simulink model "PGS_STD_SINV_2STAGE_MODEL_RLOAD"  (R2024b)
settings: Solver=VariableStepAuto  StartTime=0.0  StopTime=2.0  RelTol=1e-3
PostLoadFcn:
  | gmp_model_file=get_param(bdroot,'FileName'); if isempty(gmp_model_file), error('GMP:SINV:ModelPath', 'The SINV model must be saved before SDPE initialization.'); end; gmp_model_dir=fileparts(gmp_model_file); run(fullfile(gmp_model_dir,'sdpe_mgr','ctrl_settings_matlab_init.m')); gmp_matlab_release=matlabRelease; addpath(fullfile(gmp_model_dir,'..','..','..','..','..','slib','install_path',gmp_matlab_release.Release,'src')); clear gmp_model_file gmp_model_dir gmp_matlab_release;
InitFcn:
  | gmp_model_file=get_param(bdroot,'FileName'); if isempty(gmp_model_file), error('GMP:SINV:ModelPath', 'The SINV model must be saved before SDPE initialization.'); end; gmp_model_dir=fileparts(gmp_model_file); run(fullfile(gmp_model_dir,'sdpe_mgr','ctrl_settings_matlab_init.m')); gmp_matlab_release=matlabRelease; addpath(fullfile(gmp_model_dir,'..','..','..','..','..','slib','install_path',gmp_matlab_release.Release,'src')); clear gmp_model_file gmp_model_dir gmp_matlab_release;
undefined symbols (not defined in the file or in its folder): CTRL_AC_CURRENT_BIAS, CTRL_AC_CURRENT_SENSITIVITY, CTRL_AC_INDUCTANCE, CTRL_AC_RESISTANCE, CTRL_AC_VOLTAGE_BIAS, CTRL_AC_VOLTAGE_SENSITIVITY, CTRL_ADC_RESOLUTION, CTRL_ADC_VOLTAGE_REF, CTRL_DC_VOLTAGE_BIAS, CTRL_DC_VOLTAGE_SENSITIVITY, CTRL_DCBUS_VOLTAGE, CTRL_PWM_CMP_MAX, CTRL_PWM_DEADBAND_CMP, SINV_CURRENT_AMPLIFIER_GAIN, SINV_CURRENT_SHUNT_OHM, SINV_DC_CAP_EPR_OHM, SINV_DC_CAP_ESR_OHM, SINV_DC_CAPACITANCE_F, SINV_FILTER_CAP_EPR_OHM, SINV_FILTER_CAP_ESR_OHM, SINV_FILTER_CAPACITANCE_F, SINV_MODEL_DIODE_RON, SINV_MODEL_DIODE_VF, SINV_MODEL_MOSFET_RON, SINV_PWM_FREQUENCY_HZ, SINV_RLOAD_OHM, SINV_SENSOR_FILTER_HZ
libraries: spsSeriesRLCBranchLib x13, spsVoltageMeasurementLib x7, spsSecondOrderFilterLib x6, gmp_peripheral_utilities x3, spsMosfetLib x2, spsCurrentMeasurementLib x2, gmp_fp_utilities x1, gmp_sil_core_pack x1, spsControlledVoltageSourceLib x1, spspowerguiLib x1
(part 1 of 2)
settings Model: SimulationMode=accelerator  Creator=javnson  LastModifiedBy=javnson

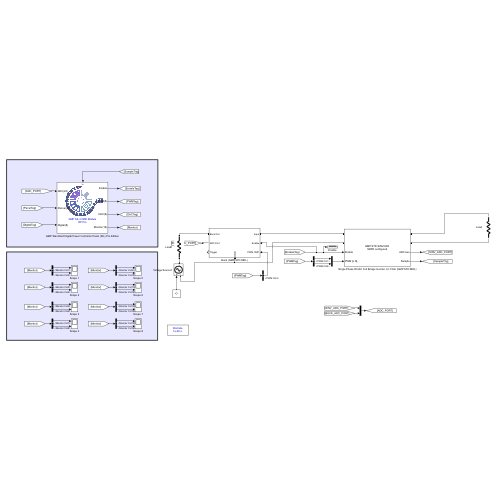
[thumbnail: Simulink's stored preview of the top-level diagram]
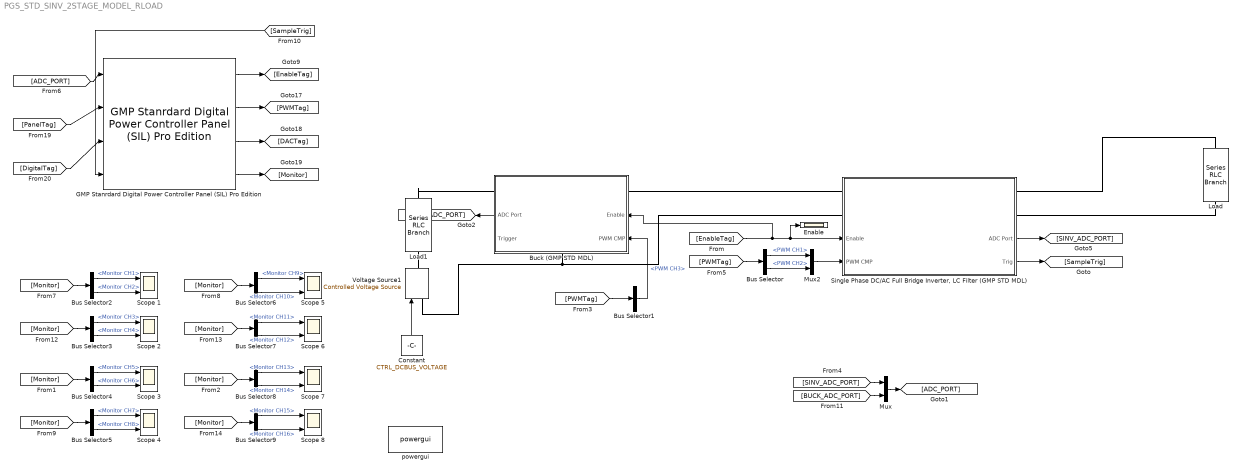
== system PGS_STD_SINV_2STAGE_MODEL_RLOAD ==
  Buck (GMP STD MDL) : Subsystem  mask(GMP Standard Digital Power Submodule - Buck){R_mosfet_on=4.6e-3, Lon=0, Rd=0.01, Vf=0.5, Rs=1e5, Cs=inf, L_main=680e-6, L_ESR=0.05, Cin_main=680e-6, Cin_ESR=0.09, Cout_main=680e-6, Cout_ESR=0.09, fswitch=20e3, CMP_MAX=4200-1, Deadband_Upper=80, Deadband_Lower=80, phase_shift=0, ADC_Resolution=12, Voltage_Gain=2.2/202.2, VOLTAGE_ADC_REFERENCE=2.5, VOLTAGE_ADC_BIAS=0.9966, VOLTAGE_ADC_INIT=0, VOLTAGE_ADC_CUT_FREQ=1.5e3, Current_Gain=0.005*20, CURRENT_ADC_REFERENCE=2.5, CURRENT_ADC_BIAS=0.9, CURRENT_ADC_INIT=0}
      mask prompts: ADC_Resolution "ADC_BIT:"; Voltage_Gain "ADC_GAIN:"; VOLTAGE_ADC_REFERENCE "ADC_REFERENCE:"; VOLTAGE_ADC_BIAS "ADC_BIAS:"; VOLTAGE_ADC_INIT "ADC_INIT:"; VOLTAGE_ADC_CUT_FREQ "cut_frequency:"; Current_Gain "ADC_GAIN:"; CURRENT_ADC_REFERENCE "ADC_REFERENCE:"; CURRENT_ADC_BIAS "ADC_BIAS:"; CURRENT_ADC_INIT "ADC_INIT:"
      mask help: This is a Standard Buck Module.
      settings: PortSchema="{\"entries\":[{\"content\":{\"sides\":[{\"content\":{\"connectorIds\":[\"LConn1\",\"In1\",\"In2\"]},\"type\":\"ConnectorPlacement.EquallySpacedRectSide\",\"uuid\":\"14f7e26c-4d08-496b-8d9c-39acdf23712e\"},{\"content\":{\"connectorIds\":[\"RConn1\",\"Out1\",\"Out2\"],\"side\":\"RIGHT\"},\"type\":\"ConnectorPlacement.EquallySpacedRectSide\",\"uuid\":\"c4fec36d-dc89-4255-810a-778c215f41bb\"},{\"content\":{\"side\":\"TOP\"},\"type\":\"ConnectorPlacement.EquallySpacedRectSide\",\"uuid\":\"1b2864bd-03e2-4902-8158-79673144629a\"},{\"content\":{\"connectorIds\":[\"RConn2\"],\"side\":\"BOTTOM\"},\"type\":\"ConnectorPlacement.EquallySpacedRectSide\",\"uuid\":\"d3456d19-e299-4c35-abfd-6fb99773e971\"}]},\"type\":\"ConnectorPlacement.EquallySpacedConnector\",\"uuid\":\"dbc738c4-c361-40e9-b3e6-9b32447065a0\"}],\"packageUris\":[\"http://schema.mathworks.com/mf0/Connector/R2020b\"],\"version\":\"1.0\"}"
      mask DialogControl ParameterGroupVar Prompt: 参数
      mask DialogControl Container4 Prompt: Component Parameters
      mask DialogControl Container7 Prompt: MOSFET
      mask DialogControl Control8 Prompt: Rds(on), unit Ohm
      mask DialogControl Control9 Prompt: Internal diode inducctance, unit H
      mask DialogControl Control10 Prompt: Internal diode resistance Rd, unit Ohm
      mask DialogControl Control11 Prompt: Internal diode forward voltage Vf, unit V
      mask DialogControl Control12 Prompt: Snubber resistance Rs, unit ohm
      mask DialogControl Control13 Prompt: Snubber Capacitance Cs, unit F
      mask DialogControl Container8 Prompt: LC Filter
      mask DialogControl Control25 Prompt: main inductance (H):
      mask DialogControl Control26 Prompt: Inductance ESR (Ohm):
      mask DialogControl Control27 Prompt: Main Input Capacitor (F):
      mask DialogControl Control28 Prompt: Input Capcitor ESR (Ohm):
      mask DialogControl Control29 Prompt: Main Output Capacitor (F):
      mask DialogControl Control30 Prompt: Output Capcitor ESR (Ohm):
      mask DialogControl Container5 Prompt: PWM Parameers
      mask DialogControl Control3 Prompt: PWM Frequency (Hz):
      mask DialogControl Control4 Prompt: Full Scale PWM Compare value:
      mask DialogControl Control6 Prompt: (whole period is 2 * CMP_MAX ticks)
      mask DialogControl Control5 Prompt: Deadband Range Set (CMP Value):
      mask DialogControl Control7 Prompt: Single side deadband time: DEADBAND_CMP/2/CMP_MAX/fswitch
      mask DialogControl Control2 Prompt: Initial Phase Shift, unit rad
      mask DialogControl Container6 Prompt: ADC Parameters
      mask DialogControl Container9 Prompt: ADC Device
      mask DialogControl Control14 Prompt: ADC resolution:
      mask DialogControl Container10 Prompt: Voltage Sensor
      mask DialogControl Control15 Prompt: ADC Voltage Gain (Scale Factor):
      mask DialogControl Control16 Prompt: ADC reference Voltage(V)
      mask DialogControl Control Prompt: ADC Bias Voltage(V)
      mask DialogControl Control18 Prompt: ADC Initial Voltage Output (V):
      mask DialogControl Control19 Prompt: Voltage Filter cut frequency (Hz):
      mask DialogControl Control20 Prompt: Generally, this value less than switch frequency / 10, greater than motor normal frequency * 3
      mask DialogControl Container11 Prompt: Current Sensor
      mask DialogControl Control21 Prompt: ADC Current Gain (Scale Factor):
      mask DialogControl Control22 Prompt: ADC reference Current(A), ADC full scale current (when gain = 1)
      mask DialogControl Control23 Prompt: ADC Bias Current(A)
      mask DialogControl Control24 Prompt: ADC initial Current Output(A)
  Bus Selector : BusSelector  OutputSignals=PWM CH1,PWM CH2
  Bus Selector1 : BusSelector  OutputSignals=PWM CH3
  Bus Selector2 : BusSelector  OutputSignals=Monitor CH1,Monitor CH2
  Bus Selector3 : BusSelector  OutputSignals=Monitor CH3,Monitor CH4
  Bus Selector4 : BusSelector  OutputSignals=Monitor CH5,Monitor CH6
  Bus Selector5 : BusSelector  OutputSignals=Monitor CH7,Monitor CH8
  Bus Selector6 : BusSelector  OutputSignals=Monitor CH9,Monitor CH10
  Bus Selector7 : BusSelector  OutputSignals=Monitor CH11,Monitor CH12
  Bus Selector8 : BusSelector  OutputSignals=Monitor CH13,Monitor CH14
  Bus Selector9 : BusSelector  OutputSignals=Monitor CH15,Monitor CH16
  Constant : Constant  Value=CTRL_DCBUS_VOLTAGE
  Enable : Scope
  GMP Stanrdard Digital Power Controller Panel (SIL) Pro Edition : gmp_sil_core_pack/GMP Stanrdard Digital Power Controller Panel (SIL) Pro Edition
      settings: SourceProductName=GMP SIL Core Utilities
  Load : spsSeriesRLCBranchLib/Series RLC Branch  LConnTagsString=__new0  RConnTagsString=__new0  BranchType=R  Resistance=SINV_RLOAD_OHM  Inductance=10e-6  SetiL0=off  InitialCurrent=0  Capacitance=1e-6  Setx0=off  InitialVoltage=0  Measurements=None
  Load1 : spsSeriesRLCBranchLib/Series RLC Branch  LConnTagsString=__new0  RConnTagsString=__new0  BranchType=R  Resistance=1  Inductance=10e-6  SetiL0=off  InitialCurrent=0  Capacitance=1e-6  Setx0=off  InitialVoltage=0  Measurements=None
  Mux : Mux  Inputs=2
  Mux2 : Mux  Inputs=2
  Scope {1..8} (8 alike) : Scope  NumInputPorts=2
  "Single Phase DC/AC Full Bridge Inverter, LC Filter (GMP STD MDL)" : Subsystem  mask(Standard Single Phase DC/AC inverter / rectifier){R_mosfet_on=SINV_MODEL_MOSFET_RON, Lon=0, Rd=SINV_MODEL_DIODE_RON, Vf=SINV_MODEL_DIODE_VF, Rs=1e5, Cs=inf, ACF_L=CTRL_AC_INDUCTANCE, ACF_L_ESR=CTRL_AC_RESISTANCE, ACF_C=SINV_FILTER_CAPACITANCE_F, ACF_C_ESR=SINV_FILTER_CAP_ESR_OHM, ACF_C_EPR=SINV_FILTER_CAP_EPR_OHM, DC_CAP=SINV_DC_CAPACITANCE_F, DC_CAP_ESR=SINV_DC_CAP_ESR_OHM, DC_CAP_EPR=SINV_DC_CAP_EPR_OHM, fswitch=SINV_PWM_FREQUENCY_HZ, CMP_MAX=CTRL_PWM_CMP_MAX + 1, Deadband_Upper=CTRL_PWM_DEADBAND_CMP, Deadband_Lower=CTRL_PWM_DEADBAND_CMP, phase_shift=0, ADC_Resolution=CTRL_ADC_RESOLUTION, DC_Voltage_Gain=CTRL_DC_VOLTAGE_SENSITIVITY, DC_VOLTAGE_ADC_REFERENCE=CTRL_ADC_VOLTAGE_REF, DC_VOLTAGE_ADC_BIAS=CTRL_DC_VOLTAGE_BIAS, DC_VOLTAGE_ADC_CUT_FREQ=SINV_SENSOR_FILTER_HZ, DC_BUS_CURRENT_SENSOR_R=SINV_CURRENT_SHUNT_OHM, DC_Current_Gain=SINV_CURRENT_AMPLIFIER_GAIN, DC_CURRENT_ADC_REFERENCE=CTRL_ADC_VOLTAGE_REF, DC_CURRENT_ADC_BIAS=CTRL_AC_CURRENT_BIAS, DC_CURRENT_ADC_CUT_FREQ=SINV_SENSOR_FILTER_HZ, AC_Voltage_Gain=CTRL_AC_VOLTAGE_SENSITIVITY, AC_VOLTAGE_ADC_REFERENCE=CTRL_ADC_VOLTAGE_REF, AC_VOLTAGE_ADC_BIAS=CTRL_AC_VOLTAGE_BIAS, AC_VOLTAGE_ADC_CUT_FREQ=SINV_SENSOR_FILTER_HZ, AC_Current_Gain=CTRL_AC_CURRENT_SENSITIVITY, AC_CURRENT_ADC_REFERENCE=CTRL_ADC_VOLTAGE_REF, AC_CURRENT_ADC_BIAS=CTRL_AC_CURRENT_BIAS, AC_CURRENT_ADC_INIT=0, CAP_CURRENT_SENSOR_R=SINV_CURRENT_SHUNT_OHM, CAP_Current_Gain=SINV_CURRENT_AMPLIFIER_GAIN, CAP_CURRENT_ADC_REFERENCE=CTRL_ADC_VOLTAGE_REF, CAP_CURRENT_ADC_BIAS=CTRL_AC_CURRENT_BIAS, CAP_CURRENT_ADC_CUT_FREQ=SINV_SENSOR_FILTER_HZ, GRID_CURRENT_SENSOR_R=SINV_CURRENT_SHUNT_OHM, Grid_Current_Gain=CTRL_AC_CURRENT_SENSITIVITY / SINV_CURRENT_SHUNT_OHM, GRID_CURRENT_ADC_REFERENCE=CTRL_ADC_VOLTAGE_REF, GRID_CURRENT_ADC_BIAS=CTRL_AC_CURRENT_BIAS, GRID_CURRENT_ADC_CUT_FREQ=SINV_SENSOR_FILTER_HZ}
      mask prompts: R_mosfet_on "MOSFET on resistance (Ohm)"; Lon "Switch series inductance (H)"; Rd "Body-diode on resistance (Ohm)"; Vf "Body-diode forward voltage (V)"; Rs "Snubber resistance (Ohm)"; Cs "Snubber capacitance (F)"; ACF_L "Series inductance (H)"; ACF_L_ESR "Series resistance (Ohm)"; ACF_C "Shunt capacitance (F)"; ACF_C_ESR "Capacitor ESR (Ohm)"; ACF_C_EPR "Capacitor leakage resistance (Ohm)"; DC_CAP "DC-link capacitance (F)"; DC_CAP_ESR "DC-link capacitor ESR (Ohm)"; DC_CAP_EPR "DC-link leakage resistance (Ohm)"; fswitch "Switching frequency (Hz)"; CMP_MAX "PWM compare full scale"; Deadband_Upper "Upper deadband (counts)"; Deadband_Lower "Lower deadband (counts)"; phase_shift "Carrier phase shift (deg)"; ADC_Resolution "ADC resolution (bits)"; DC_Voltage_Gain "DC voltage sensitivity (V/V)"; DC_VOLTAGE_ADC_REFERENCE "DC voltage ADC reference (V)"; DC_VOLTAGE_ADC_BIAS "DC voltage ADC bias (V)"; DC_VOLTAGE_ADC_CUT_FREQ "DC voltage filter cutoff (Hz)"; DC_BUS_CURRENT_SENSOR_R "DC shunt resistance (Ohm)"; DC_Current_Gain "DC current amplifier gain"; DC_CURRENT_ADC_REFERENCE "DC current ADC reference (V)"; DC_CURRENT_ADC_BIAS "DC current ADC bias (V)"; DC_CURRENT_ADC_CUT_FREQ "DC current filter cutoff (Hz)"; AC_Voltage_Gain "AC voltage sensitivity (V/V)"; AC_VOLTAGE_ADC_REFERENCE "AC voltage ADC reference (V)"; AC_VOLTAGE_ADC_BIAS "AC voltage ADC bias (V)"; AC_VOLTAGE_ADC_CUT_FREQ "AC voltage filter cutoff (Hz)"; AC_Current_Gain "AC current sensitivity (V/A)"; AC_CURRENT_ADC_REFERENCE "AC current ADC reference (V)"; AC_CURRENT_ADC_BIAS "AC current ADC bias (V)"; AC_CURRENT_ADC_INIT "AC current initial value"; CAP_CURRENT_SENSOR_R "Capacitor-current shunt (Ohm)"; CAP_Current_Gain "Capacitor-current amplifier gain"; CAP_CURRENT_ADC_REFERENCE "Capacitor-current ADC reference (V)"; CAP_CURRENT_ADC_BIAS "Capacitor-current ADC bias (V)"; CAP_CURRENT_ADC_CUT_FREQ "Capacitor-current filter cutoff (Hz)"; GRID_CURRENT_SENSOR_R "Grid-current shunt (Ohm)"; Grid_Current_Gain "Grid-current amplifier gain"; GRID_CURRENT_ADC_REFERENCE "Grid-current ADC reference (V)"; GRID_CURRENT_ADC_BIAS "Grid-current ADC bias (V)"; GRID_CURRENT_ADC_CUT_FREQ "Grid-current filter cutoff (Hz)"
      mask help: SDPE-configured single-phase bidirectional converter. ADC bus order: IL, IDC, VDC, IC, VC, IG. PWM order: bridge legs L and N.
      settings: PortSchema="{\"entries\":[{\"content\":{\"sides\":[{\"content\":{\"connectorIds\":[\"LConn1\",\"LConn2\",\"In1\",\"In2\"]},\"type\":\"ConnectorPlacement.EquallySpacedRectSide\",\"uuid\":\"0e3e6e75-5e1a-455b-8a22-c69d0a4261ca\"},{\"content\":{\"connectorIds\":[\"RConn1\",\"RConn2\",\"Out1\",\"Out2\"],\"side\":\"RIGHT\"},\"type\":\"ConnectorPlacement.EquallySpacedRectSide\",\"uuid\":\"20326781-9238-4fea-80fd-ba96906d5d3f\"},{\"content\":{\"side\":\"TOP\"},\"type\":\"ConnectorPlacement.EquallySpacedRectSide\",\"uuid\":\"9e3289d3-0bee-4337-807b-c293a46cda9c\"}]},\"type\":\"ConnectorPlacement.EquallySpacedConnector\",\"uuid\":\"56bb35ad-d602-4874-b9bf-b95a81ef662c\"}],\"packageUris\":[\"http://schema.mathworks.com/mf0/Connector/R2020b\"],\"version\":\"1.0\"}"
      mask DialogControl ParameterGroupVar Prompt: 参数
      mask DialogControl Container4 Prompt: Component Parameters
      mask DialogControl Container7 Prompt: MOSFET
      mask DialogControl Control2 Prompt: Rds(on), unit Ohm
      mask DialogControl Control3 Prompt: Internal diode inducctance, unit H
      mask DialogControl Control4 Prompt: Internal diode resistance Rd, unit Ohm
      mask DialogControl Control5 Prompt: Internal diode forward voltage Vf, unit V
      mask DialogControl Control6 Prompt: Snubber resistance Rs, unit ohm
      mask DialogControl Control7 Prompt: Snubber Capacitance Cs, unit F
      mask DialogControl Container8 Prompt: LC Filter
      mask DialogControl Container20 Prompt: Filter Inductor
      mask DialogControl Control8 Prompt: AC Bus Filter Inductor (H)
      mask DialogControl Control42 Prompt: AC Bus Filter Inductor, ESR (Ohm)
      mask DialogControl Container21 Prompt: Filter Capcitor
      mask DialogControl Control43 Prompt: AC Bus Filter Capacitor (F)
      mask DialogControl Control44 Prompt: AC Bus Filter Capacitor, ESR (Ohm)
      mask DialogControl Control45 Prompt: AC Bus Filter Capacitor, EPR (Ohm)
      mask DialogControl Container22 Prompt: DC Bus Capacitor
      mask DialogControl Control46 Prompt: DC Bus Capacitor (F)
      mask DialogControl Control47 Prompt: DC Bus Capacitor, ESR (Ohm)
      mask DialogControl Control48 Prompt: DC Bus Capacitor, EPR (Ohm)
      mask DialogControl Container5 Prompt: PWM Parameers
      mask DialogControl Control9 Prompt: PWM Frequency (Hz):
      mask DialogControl Control10 Prompt: Full Scale PWM Compare value:
      mask DialogControl Control11 Prompt: (whole period is 2 * CMP_MAX ticks)
      mask DialogControl Control12 Prompt: Deadband Range Set (CMP Value):
      mask DialogControl Control13 Prompt: Single side deadband time: DEADBAND_CMP/2/CMP_MAX/fswitch
      mask DialogControl Control14 Prompt: Initial Phase Shift, unit rad
      mask DialogControl Container6 Prompt: ADC Parameters
      mask DialogControl Container14 Prompt: ADC Device
      mask DialogControl Control15 Prompt: ADC resolution:
      mask DialogControl Container15 Prompt: DC Side Voltage Sensor
      mask DialogControl Control16 Prompt: ADC Voltage Gain (Scale Factor):
      mask DialogControl Control17 Prompt: ADC reference Voltage(V)
      mask DialogControl Control18 Prompt: ADC Bias Voltage(V)
      mask DialogControl Control19 Prompt: Voltage Filter cut frequency (Hz):
      mask DialogControl Control20 Prompt: Generally, this value less than switch frequency / 10, greater than motor normal frequency * 3
      mask DialogControl Container16 Prompt: DC Side Current Sensor
      mask DialogControl Control26 Prompt: DC Bus Current Sensor Resistance
      mask DialogControl Control34 Prompt: ADC Current Gain (Scale Factor):
      mask DialogControl Control27 Prompt: ADC reference Voltage(V), ADC full scale current (when gain = 1)
      mask DialogControl Control28 Prompt: ADC Bias Current(A)
      mask DialogControl Control35 Prompt: Voltage Filter cut frequency (Hz):
      mask DialogControl Control36 Prompt: Generally, this value less than switch frequency / 10, greater than motor normal frequency * 3
      mask DialogControl Container17 Prompt: AC Side Voltage Sensor
      mask DialogControl Control16_copy Prompt: ADC Voltage Gain (Scale Factor):
      mask DialogControl Control17_copy Prompt: ADC reference Voltage(V)
      mask DialogControl Control18_copy Prompt: ADC Bias Voltage(V)
      mask DialogControl Control19_copy Prompt: Voltage Filter cut frequency (Hz):
      mask DialogControl Control20_copy Prompt: Generally, this value less than switch frequency / 10, greater than motor normal frequency * 3
      mask DialogControl Container18 Prompt: AC Side Current Sensor
      mask DialogControl Control26_copy Prompt: ADC Current Gain (Scale Factor):
      mask DialogControl Control27_copy Prompt: ADC reference Current(A), ADC full scale current (when gain = 1)
      mask DialogControl Control28_copy Prompt: ADC Bias Current(A)
      mask DialogControl Control29_copy Prompt: ADC initial Current Output(A)
      mask DialogControl Container19 Prompt: Capcitor Current Sensor
      mask DialogControl Control26_copy_copy Prompt: Filter Capacitor Current Sensor Resistance
      mask DialogControl Control34_copy Prompt: ADC Current Gain (Scale Factor):
      mask DialogControl Control27_copy_copy Prompt: ADC reference Voltage(V), ADC full scale current (when gain = 1)
      mask DialogControl Control28_copy_copy Prompt: ADC Bias Current(V)
      mask DialogControl Control35_copy Prompt: Voltage Filter cut frequency (Hz):
      mask DialogControl Control36_copy Prompt: Generally, this value less than switch frequency / 10, greater than motor normal frequency * 3
      mask DialogControl Container23 Prompt: Grid Current Sensor
      mask DialogControl Control26_copy_copy_copy Prompt: Grid Bus Current Sensor Resistance
      mask DialogControl Control34_copy_copy Prompt: ADC Current Gain (Scale Factor):
      mask DialogControl Control27_copy_copy_copy Prompt: ADC reference Voltage(V), ADC full scale current (when gain = 1)
      mask DialogControl Control28_copy_copy_copy Prompt: ADC Bias Current(V)
      mask DialogControl Control35_copy_copy Prompt: Voltage Filter cut frequency (Hz):
      mask DialogControl Control36_copy_copy Prompt: Generally, this value less than switch frequency / 10, greater than motor normal frequency * 3
      mask DialogControl PWMConfiguration_Group Prompt: PWM Configuration
      mask DialogControl SemiconductorModel_Group Prompt: Semiconductor Model
      mask DialogControl ACFilter_Group Prompt: AC Filter
      mask DialogControl DCLink_Group Prompt: DC Link
      mask DialogControl ADCConfiguration_Group Prompt: ADC Configuration
      mask DialogControl VoltageSensors_Group Prompt: Voltage Sensors
      mask DialogControl CurrentSensors_Group Prompt: Current Sensors
      mask Display:
      | disp('GMP STD SINV/AFE\nSDPE configured');
      | port_label('input',1,'Enable'); port_label('input',2,'PWM [L N]');
      | port_label('output',1,'ADC bus'); port_label('output',2,'Sample');
  Voltage Source1 : spsControlledVoltageSourceLib/Controlled Voltage Source  Initialize=on  Source_Type=AC  Amplitude=0  Phase=0  Frequency=0  Measurements=None
  powergui : spspowerguiLib/powergui  Priority=1  SimulationMode=Discrete  SampleTime=1e-6  frequency=60  Iterations=50  frequencyindice=0  Pbase=100e6  ErrMax=1e-4  UnitsV=kV  UnitsW=MW  buscounter=0  FunctionMessages=off  echomessages=off  EnableUseOfTLC=off  CurrentSourceSwitches=off  DisableSnubberDevices=off  DisableRonSwitches=off  DisableVfSwitches=off  DisplayEquations=off  AutomaticDiscreteSolvers=off  SolverType=Tustin/Backward Euler (TBE)  Interpol=off  ExternalGateDelay=off  methode=off  Ts=100  x0status=blocks  SPID=on  SwTol=0  HookPort=off  NonlinearTolerance=1e-4  nMaxIteration=100  ContinueOnMaxIteration=off  RestoreLinks=warning  ResistiveCurrentMeasurement=off  Frange=[0:2:500]  Ylog=off  Xlog=on  ShowGrid=off  save=off  variable=ZData  structure=0  ZoomFFT=off  StartTime=0.0  cycles=1  DisplayStyle=1  fundamental=60  FreqAxis=off  MaxFrequency=1000  frequencyindicesteady=1  RmsSteady=1  display=off
  wires:
  [PanelTag] -> GMP Stanrdard Digital Power Controller Panel (SIL) Pro Edition/2
  [SampleTrig] -> GMP Stanrdard Digital Power Controller Panel (SIL) Pro Edition/4
  GMP Stanrdard Digital Power Controller Panel (SIL) Pro Edition/2 -> [PWMTag]
  [ADC_PORT] -> GMP Stanrdard Digital Power Controller Panel (SIL) Pro Edition/1
  GMP Stanrdard Digital Power Controller Panel (SIL) Pro Edition/4 -> [Monitor]
  GMP Stanrdard Digital Power Controller Panel (SIL) Pro Edition/1 -> [EnableTag]
  GMP Stanrdard Digital Power Controller Panel (SIL) Pro Edition/3 -> [DACTag]
  [DigitalTag] -> GMP Stanrdard Digital Power Controller Panel (SIL) Pro Edition/3
  [EnableTag] -> Buck (GMP STD MDL)/1(Enable), "Single Phase DC/AC Full Bridge Inverter, LC Filter (GMP STD MDL)"/1(Enable), Enable/1
  Bus Selector8/2 -> Scope 7/2  "<Monitor CH14>"
  Bus Selector2/2 -> Scope 1/2  "<Monitor CH2>"
  Bus Selector4/2 -> Scope 3/2  "<Monitor CH6>"
  Bus Selector3/1 -> Scope 2/1  "<Monitor CH3>"
  [Monitor] -> Bus Selector4/1
  [Monitor] -> Bus Selector7/1
  Bus Selector2/1 -> Scope 1/1  "<Monitor CH1>"
  Bus Selector5/1 -> Scope 4/1  "<Monitor CH7>"
  [Monitor] -> Bus Selector3/1
  Bus Selector8/1 -> Scope 7/1  "<Monitor CH13>"
  Bus Selector3/2 -> Scope 2/2  "<Monitor CH4>"
  Bus Selector4/1 -> Scope 3/1  "<Monitor CH5>"
  Bus Selector7/1 -> Scope 6/1  "<Monitor CH11>"
  [Monitor] -> Bus Selector5/1
  [Monitor] -> Bus Selector8/1
  [Monitor] -> Bus Selector6/1
  Bus Selector6/1 -> Scope 5/1  "<Monitor CH9>"
  Bus Selector5/2 -> Scope 4/2  "<Monitor CH8>"
  [Monitor] -> Bus Selector2/1
  Bus Selector7/2 -> Scope 6/2  "<Monitor CH12>"
  Bus Selector6/2 -> Scope 5/2  "<Monitor CH10>"
  Bus Selector/1 -> Mux2/1  "<PWM CH1>"
  [PWMTag] -> Bus Selector/1
  Bus Selector9/1 -> Scope 8/1  "<Monitor CH15>"
  [Monitor] -> Bus Selector9/1
  Bus Selector9/2 -> Scope 8/2  "<Monitor CH16>"
  "Single Phase DC/AC Full Bridge Inverter, LC Filter (GMP STD MDL)"/1(ADC Port) -> [SINV_ADC_PORT]
  "Single Phase DC/AC Full Bridge Inverter, LC Filter (GMP STD MDL)"/2(Trig) -> [SampleTrig]
  Bus Selector/2 -> Mux2/2  "<PWM CH2>"
  Mux2/1 -> "Single Phase DC/AC Full Bridge Inverter, LC Filter (GMP STD MDL)"/2(PWM CMP)
  Constant/1 -> Voltage Source1/1
  [PWMTag] -> Bus Selector1/1
  Bus Selector1/1 -> Buck (GMP STD MDL)/2(PWM CMP)  "<PWM CH3>"
  Buck (GMP STD MDL)/1(ADC Port) -> [BUCK_ADC_PORT]
  Mux/1 -> [ADC_PORT]
  [SINV_ADC_PORT] -> Mux/1
  [BUCK_ADC_PORT] -> Mux/2
  connections:
  Load/LConn1 -- "Single Phase DC/AC Full Bridge Inverter, LC Filter (GMP STD MDL)"/RConn1
  Load/RConn1 -- "Single Phase DC/AC Full Bridge Inverter, LC Filter (GMP STD MDL)"/RConn2
  Voltage Source1/RConn1 -- Load1/RConn1
  Buck (GMP STD MDL)/LConn1 -- "Single Phase DC/AC Full Bridge Inverter, LC Filter (GMP STD MDL)"/LConn1
  "Single Phase DC/AC Full Bridge Inverter, LC Filter (GMP STD MDL)"/LConn2 -- Voltage Source1/LConn1 -- Buck (GMP STD MDL)/RConn2
  Load1/LConn1 -- Buck (GMP STD MDL)/RConn1

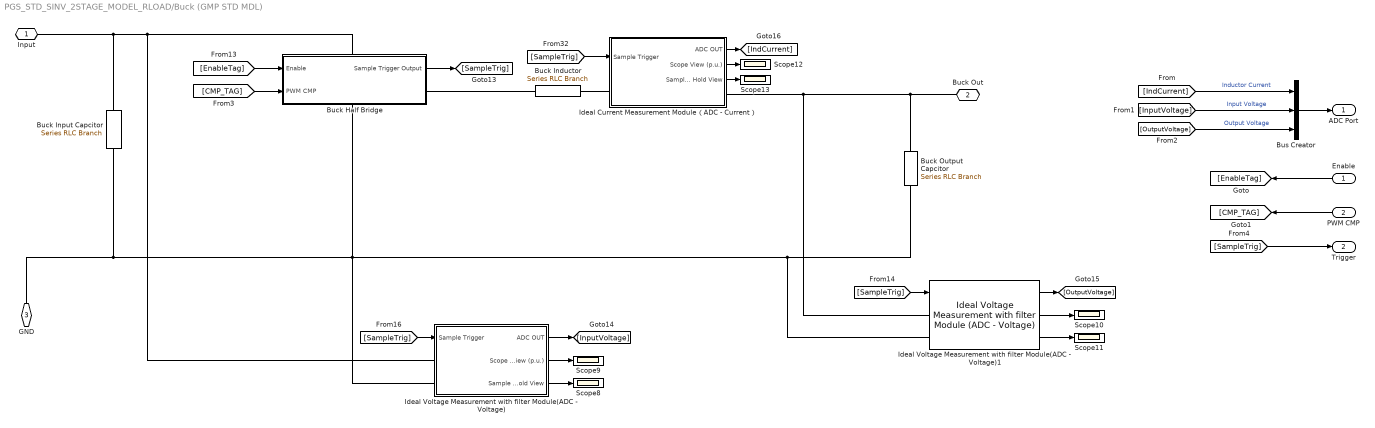
== system PGS_STD_SINV_2STAGE_MODEL_RLOAD/Buck (GMP STD MDL) ==
  Enable : Inport
  PWM CMP : Inport  Port=2
  Buck Half Bridge : Subsystem  mask{fswitch=fswitch, CMP_MAX=CMP_MAX, Deadband_Upper=Deadband_Upper, Deadband_Lower=Deadband_Lower, Deadband_us=NaN, phase_shift=phase_shift, R_mosfet_on=R_mosfet_on, Lon=Lon, Rd=Rd, Vf=Vf, Rs=Rs, Cs=Cs}
      mask init:
      | calculate_deadband(gcb, 'Deadband_Upper', 'Deadband_Lower',	'CMP_MAX', 'fswitch', 'Deadband_us');
      settings: PortSchema="{\"entries\":[{\"content\":{\"sides\":[{\"content\":{\"connectorIds\":[\"In1\",\"In2\"]},\"type\":\"ConnectorPlacement.EquallySpacedRectSide\",\"uuid\":\"20beeabc-b0ca-4337-b227-c7f02abd15d8\"},{\"content\":{\"connectorIds\":[\"Out1\",\"RConn1\"],\"side\":\"RIGHT\"},\"type\":\"ConnectorPlacement.EquallySpacedRectSide\",\"uuid\":\"a7923383-ac55-4621-ad1d-4d067c1fb84d\"},{\"content\":{\"connectorIds\":[\"LConn1\"],\"side\":\"TOP\"},\"type\":\"ConnectorPlacement.EquallySpacedRectSide\",\"uuid\":\"661bf0ae-1c96-4de8-96aa-28c06a0a56db\"},{\"content\":{\"connectorIds\":[\"RConn2\"],\"side\":\"BOTTOM\"},\"type\":\"ConnectorPlacement.EquallySpacedRectSide\",\"uuid\":\"fc2f6321-5787-4e1a-b5a2-65ed34db36b5\"}]},\"type\":\"ConnectorPlacement.EquallySpacedConnector\",\"uuid\":\"e2219b16-0a50-43ef-8183-c55a35d5a2a0\"}],\"packageUris\":[\"http://schema.mathworks.com/mf0/Connector/R2020b\"],\"version\":\"1.0\"}"
      mask Callback fswitch: calculate_deadband(gcb, 'Deadband_Upper', 'Deadband_Lower',	'CMP_MAX', 'fswitch', 'Deadband_us');
      mask Callback CMP_MAX: calculate_deadband(gcb, 'Deadband_Upper', 'Deadband_Lower',	'CMP_MAX', 'fswitch', 'Deadband_us');
      mask Callback Deadband_Upper: calculate_deadband(gcb, 'Deadband_Upper', 'Deadband_Lower',	'CMP_MAX', 'fswitch', 'Deadband_us');
      mask Callback Deadband_Lower: calculate_deadband(gcb, 'Deadband_Upper', 'Deadband_Lower',	'CMP_MAX', 'fswitch', 'Deadband_us');
      mask DialogControl DescGroupVar Prompt: Half Bridge With PWM Module
      mask DialogControl Control14 Prompt: GMP CTL Simulink Utilities: virtual peripherals
      mask DialogControl DescTextVar Prompt: This module provide a PWM (with deadband), and a MOSFET half bridge.
      mask DialogControl Container5 Prompt: PWM Modulator
      mask DialogControl ParameterGroupVar Prompt: PWM module parameters
      mask DialogControl Control2 Prompt: PWM Frequency (Hz):
      mask DialogControl Control3 Prompt: Full Scale PWM Compare value:
      mask DialogControl Control4 Prompt: (whole period is 2 * CMP_MAX ticks)
      mask DialogControl Control5 Prompt: Deadband Range Set (CMP Value):
      mask DialogControl Control6 Prompt: Single side deadband time: DEADBAND_CMP/2/CMP_MAX/fswitch
      mask DialogControl Control15 Prompt: Calculated Deadband, us
      mask DialogControl Control13 Prompt: Initial Phase Shift, unit rad
      mask DialogControl Container6 Prompt: MOSFET
      mask DialogControl Container3 Prompt: MOSFET parameters
      mask DialogControl Control7 Prompt: Rds(on), unit Ohm
      mask DialogControl Control8 Prompt: Internal diode inducctance, unit H
      mask DialogControl Control9 Prompt: Internal diode resistance Rd, unit Ohm
      mask DialogControl Control10 Prompt: Internal diode forward voltage Vf, unit V
      mask DialogControl Control11 Prompt: Snubber resistance Rs, unit ohm
      mask DialogControl Control12 Prompt: Snubber Capacitance Cs, unit F
  Buck Inductor : spsSeriesRLCBranchLib/Series RLC Branch  LConnTagsString=__new0  RConnTagsString=__new0  BranchType=RL  Resistance=L_ESR  Inductance=L_main  SetiL0=off  InitialCurrent=0  Capacitance=1e-6  Setx0=off  InitialVoltage=0  Measurements=None
  Buck Input Capcitor : spsSeriesRLCBranchLib/Series RLC Branch  LConnTagsString=__new0  RConnTagsString=__new0  BranchType=RC  Resistance=Cin_ESR  Inductance=1e-3  SetiL0=off  InitialCurrent=0  Capacitance=Cin_main  Setx0=off  InitialVoltage=0  Measurements=None
  Buck Output Capcitor : spsSeriesRLCBranchLib/Series RLC Branch  LConnTagsString=__new0  RConnTagsString=__new0  BranchType=RC  Resistance=Cout_ESR  Inductance=1e-3  SetiL0=off  InitialCurrent=0  Capacitance=Cout_main  Setx0=off  InitialVoltage=0  Measurements=None
  Bus Creator : BusCreator  Inputs=3
  Ideal Current Measurement Module（ADC - Current） : Subsystem  mask{ADC_GAIN=Current_Gain, ADC_BIT=ADC_Resolution, ADC_REFERENCE=CURRENT_ADC_REFERENCE, ADC_BIAS=CURRENT_ADC_BIAS, ADC_INIT=CURRENT_ADC_INIT}
      mask DialogControl DescGroupVar Prompt: Current Sample ADC Model 1
      mask DialogControl DescTextVar Prompt: This is a ideal Current Measurement Module. This module enable a bias and a gain, and finally output a ADC result.
      mask DialogControl Control8 Prompt: ADC(p.u.) = (real_current * ADC_GAIN + ADC_BIAS)/ADC_REFERENCE
      mask DialogControl Control9 Prompt: GMP CTL Simulink Utilities: virtual peripherals
      mask DialogControl ParameterGroupVar Prompt: 参数
      mask DialogControl Control7 Prompt: ADC Current Gain (Scale Factor):
      mask DialogControl Control2 Prompt: ADC resolution:
      mask DialogControl Control4 Prompt: ADC reference Current(A), ADC full scale current (when gain = 1)
      mask DialogControl Control5 Prompt: ADC Bias Current(A)
      mask DialogControl Control6 Prompt: ADC initial Current Output(A)
  Ideal Voltage Measurement with filter Module(ADC - Voltage) : Subsystem  mask{ADC_GAIN=Voltage_Gain, ADC_BIT=ADC_Resolution, ADC_REFERENCE=VOLTAGE_ADC_REFERENCE, ADC_BIAS=VOLTAGE_ADC_BIAS, ADC_INIT=VOLTAGE_ADC_INIT, cut_frequency=VOLTAGE_ADC_CUT_FREQ}
      mask DialogControl DescGroupVar Prompt: Voltage Sample ADC Model
      mask DialogControl DescTextVar Prompt: This is a ideal Voltage Measurement Module.
      mask DialogControl Control2 Prompt: ADC(p.u.) = (real_voltage * ADC_GAIN + ADC_BIAS)/ADC_REFERENCE
      mask DialogControl Control11 Prompt: GMP CTL Simulink Utilities: virtual peripherals
      mask DialogControl ParameterGroupVar Prompt: Parameters:
      mask DialogControl Control4 Prompt: ADC Voltage Gain (Scale Factor):
      mask DialogControl Control5 Prompt: ADC resolution:
      mask DialogControl Control6 Prompt: ADC reference Voltage(V)
      mask DialogControl Control8 Prompt: ADC Bias Voltage(V)
      mask DialogControl Control7 Prompt: ADC Initial Voltage Output (V):
      mask DialogControl Control9 Prompt: Voltage Filter cut frequency (Hz):
      mask DialogControl Control10 Prompt: Generally, this value less than switch frequency / 10, greater than motor normal frequency * 3
  Ideal Voltage Measurement with filter Module(ADC - Voltage)1 : gmp_peripheral_utilities/Ideal Voltage Measurement with filter Module (ADC - Voltage)  ADC_GAIN=Voltage_Gain  ADC_BIT=ADC_Resolution  ADC_REFERENCE=VOLTAGE_ADC_REFERENCE  ADC_BIAS=VOLTAGE_ADC_BIAS  ADC_INIT=VOLTAGE_ADC_INIT  cut_frequency=VOLTAGE_ADC_CUT_FREQ
      settings: SourceProductName=Virtual Peripheral Utilities
  Scope{8..13} (6 alike) : Scope
  Input : PMIOPort  Side=Left
  Buck Out : PMIOPort  Port=2  Side=Right
  GND : PMIOPort  Port=3  Side=Right
  ADC Port : Outport
  Trigger : Outport  Port=2
  wires:
  [InputVoltage] -> Bus Creator/2  "Input Voltage"
  [SampleTrig] -> Trigger/1
  PWM CMP/1 -> [CMP_TAG]
  Enable/1 -> [EnableTag]
  Bus Creator/1 -> ADC Port/1
  [OutputVoltage] -> Bus Creator/3  "Output Voltage"
  [IndCurrent] -> Bus Creator/1  "Inductor Current"
  [CMP_TAG] -> Buck Half Bridge/2(PWM CMP)
  Ideal Current Measurement Module（ADC - Current）/1(ADC OUT) -> [IndCurrent]
  Ideal Voltage Measurement with filter Module(ADC - Voltage)/1(ADC OUT) -> [InputVoltage]
  Ideal Voltage Measurement with filter Module(ADC - Voltage)1/1 -> [OutputVoltage]
  Ideal Voltage Measurement with filter Module(ADC - Voltage)/2(Scope View (p.u.)) -> Scope9/1
  Ideal Voltage Measurement with filter Module(ADC - Voltage)1/3 -> Scope11/1
  Ideal Voltage Measurement with filter Module(ADC - Voltage)/3(Sample & Hold View) -> Scope8/1
  [SampleTrig] -> Ideal Current Measurement Module（ADC - Current）/1(Sample Trigger)
  Buck Half Bridge/1(Sample Trigger Output) -> [SampleTrig]
  Ideal Current Measurement Module（ADC - Current）/3(Sample & Hold View) -> Scope13/1
  Ideal Current Measurement Module（ADC - Current）/2(Scope View (p.u.)) -> Scope12/1
  [EnableTag] -> Buck Half Bridge/1(Enable)
  Ideal Voltage Measurement with filter Module(ADC - Voltage)1/2 -> Scope10/1
  [SampleTrig] -> Ideal Voltage Measurement with filter Module(ADC - Voltage)1/1
  [SampleTrig] -> Ideal Voltage Measurement with filter Module(ADC - Voltage)/1(Sample Trigger)
  connections:
  Buck Half Bridge/RConn1 -- Buck Inductor/LConn1
  Ideal Voltage Measurement with filter Module(ADC - Voltage)/LConn1 -- Buck Half Bridge/LConn1 -- Input/RConn1 -- Buck Input Capcitor/LConn1
  Buck Out/RConn1 -- Buck Output Capcitor/LConn1 -- Ideal Voltage Measurement with filter Module(ADC - Voltage)1/LConn1 -- Ideal Current Measurement Module（ADC - Current）/RConn1
  GND/RConn1 -- Buck Input Capcitor/RConn1 -- Buck Half Bridge/RConn2 -- Ideal Voltage Measurement with filter Module(ADC - Voltage)/LConn2 -- Buck Output Capcitor/RConn1 -- Ideal Voltage Measurement with filter Module(ADC - Voltage)1/LConn2
  Ideal Current Measurement Module（ADC - Current）/LConn1 -- Buck Inductor/RConn1

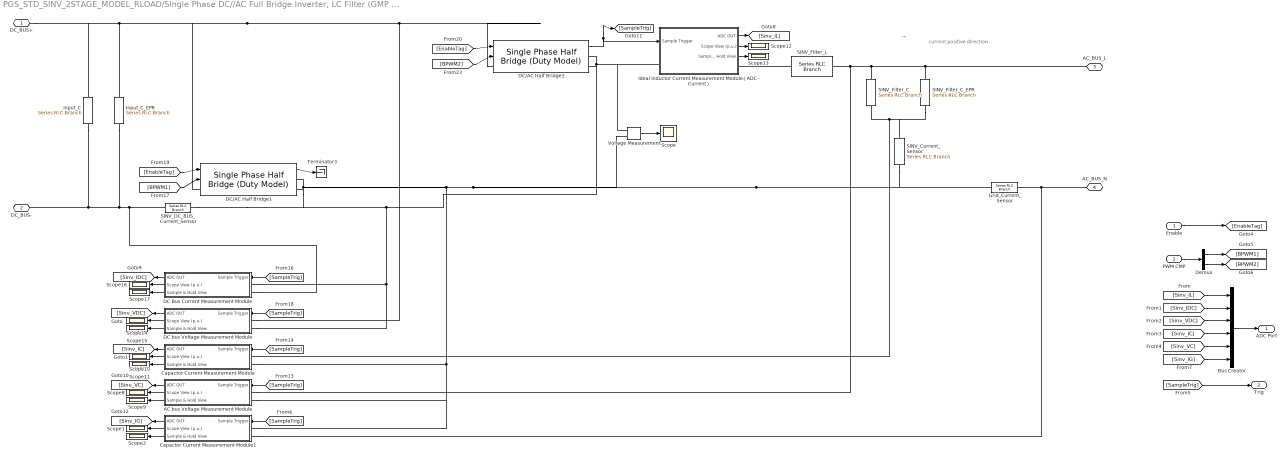
== system PGS_STD_SINV_2STAGE_MODEL_RLOAD/Single Phase DC//AC Full Bridge Inverter, LC Filter (GMP STD MDL) ==
  note: →
  note: current positive direction
  Enable : Inport
  PWM CMP : Inport  Port=2
  AC bus Voltage Measurement Module : Subsystem  AncestorBlock=peripheral_utilities/Ideal Voltage Measurement with filter Module(ADC - Voltage)  mask{ADC_GAIN=AC_Voltage_Gain, ADC_BIT=ADC_Resolution, ADC_REFERENCE=AC_VOLTAGE_ADC_REFERENCE, ADC_BIAS=AC_VOLTAGE_ADC_BIAS, ADC_INIT=0, cut_frequency=AC_VOLTAGE_ADC_CUT_FREQ}
      mask DialogControl DescGroupVar Prompt: Voltage Sample ADC Model
      mask DialogControl DescTextVar Prompt: This is a ideal Voltage Measurement Module.
      mask DialogControl Control2 Prompt: ADC(p.u.) = (real_voltage * ADC_GAIN + ADC_BIAS)/ADC_REFERENCE
      mask DialogControl Control11 Prompt: GMP CTL Simulink Utilities: virtual peripherals
      mask DialogControl ParameterGroupVar Prompt: Parameters:
      mask DialogControl Control4 Prompt: ADC Voltage Gain (Scale Factor):
      mask DialogControl Control5 Prompt: ADC resolution:
      mask DialogControl Control6 Prompt: ADC reference Voltage(V)
      mask DialogControl Control8 Prompt: ADC Bias Voltage(V)
      mask DialogControl Control7 Prompt: ADC Initial Voltage Output (V):
      mask DialogControl Control9 Prompt: Voltage Filter cut frequency (Hz):
      mask DialogControl Control10 Prompt: Generally, this value less than switch frequency / 10, greater than motor normal frequency * 3
  Bus Creator : BusCreator  Inputs=6
  Capactor Current Measurement Module : Subsystem  AncestorBlock=peripheral_utilities/Ideal Voltage Measurement with filter Module(ADC - Voltage)  mask{ADC_GAIN=CAP_Current_Gain, ADC_BIT=ADC_Resolution, ADC_REFERENCE=CAP_CURRENT_ADC_REFERENCE, ADC_BIAS=CAP_CURRENT_ADC_BIAS, ADC_INIT=0, cut_frequency=CAP_CURRENT_ADC_CUT_FREQ}
      mask DialogControl DescGroupVar Prompt: Voltage Sample ADC Model
      mask DialogControl DescTextVar Prompt: This is a ideal Voltage Measurement Module.
      mask DialogControl Control2 Prompt: ADC(p.u.) = (real_voltage * ADC_GAIN + ADC_BIAS)/ADC_REFERENCE
      mask DialogControl Control11 Prompt: GMP CTL Simulink Utilities: virtual peripherals
      mask DialogControl ParameterGroupVar Prompt: Parameters:
      mask DialogControl Control4 Prompt: ADC Voltage Gain (Scale Factor):
      mask DialogControl Control5 Prompt: ADC resolution:
      mask DialogControl Control6 Prompt: ADC reference Voltage(V)
      mask DialogControl Control8 Prompt: ADC Bias Voltage(V)
      mask DialogControl Control7 Prompt: ADC Initial Voltage Output (V):
      mask DialogControl Control9 Prompt: Voltage Filter cut frequency (Hz):
      mask DialogControl Control10 Prompt: Generally, this value less than switch frequency / 10, greater than motor normal frequency * 3
  Capactor Current Measurement Module1 : Subsystem  AncestorBlock=peripheral_utilities/Ideal Voltage Measurement with filter Module(ADC - Voltage)  mask{ADC_GAIN=Grid_Current_Gain, ADC_BIT=ADC_Resolution, ADC_REFERENCE=GRID_CURRENT_ADC_REFERENCE, ADC_BIAS=GRID_CURRENT_ADC_BIAS, ADC_INIT=0, cut_frequency=GRID_CURRENT_ADC_CUT_FREQ}
      mask DialogControl DescGroupVar Prompt: Voltage Sample ADC Model
      mask DialogControl DescTextVar Prompt: This is a ideal Voltage Measurement Module.
      mask DialogControl Control2 Prompt: ADC(p.u.) = (real_voltage * ADC_GAIN + ADC_BIAS)/ADC_REFERENCE
      mask DialogControl Control11 Prompt: GMP CTL Simulink Utilities: virtual peripherals
      mask DialogControl ParameterGroupVar Prompt: Parameters:
      mask DialogControl Control4 Prompt: ADC Voltage Gain (Scale Factor):
      mask DialogControl Control5 Prompt: ADC resolution:
      mask DialogControl Control6 Prompt: ADC reference Voltage(V)
      mask DialogControl Control8 Prompt: ADC Bias Voltage(V)
      mask DialogControl Control7 Prompt: ADC Initial Voltage Output (V):
      mask DialogControl Control9 Prompt: Voltage Filter cut frequency (Hz):
      mask DialogControl Control10 Prompt: Generally, this value less than switch frequency / 10, greater than motor normal frequency * 3
  DC Bus Current Measurement Module : Subsystem  AncestorBlock=peripheral_utilities/Ideal Voltage Measurement with filter Module(ADC - Voltage)  mask{ADC_GAIN=DC_Current_Gain, ADC_BIT=ADC_Resolution, ADC_REFERENCE=DC_CURRENT_ADC_REFERENCE, ADC_BIAS=DC_CURRENT_ADC_BIAS, ADC_INIT=0, cut_frequency=DC_CURRENT_ADC_CUT_FREQ}
      mask DialogControl DescGroupVar Prompt: Voltage Sample ADC Model
      mask DialogControl DescTextVar Prompt: This is a ideal Voltage Measurement Module.
      mask DialogControl Control2 Prompt: ADC(p.u.) = (real_voltage * ADC_GAIN + ADC_BIAS)/ADC_REFERENCE
      mask DialogControl Control11 Prompt: GMP CTL Simulink Utilities: virtual peripherals
      mask DialogControl ParameterGroupVar Prompt: Parameters:
      mask DialogControl Control4 Prompt: ADC Voltage Gain (Scale Factor):
      mask DialogControl Control5 Prompt: ADC resolution:
      mask DialogControl Control6 Prompt: ADC reference Voltage(V)
      mask DialogControl Control8 Prompt: ADC Bias Voltage(V)
      mask DialogControl Control7 Prompt: ADC Initial Voltage Output (V):
      mask DialogControl Control9 Prompt: Voltage Filter cut frequency (Hz):
      mask DialogControl Control10 Prompt: Generally, this value less than switch frequency / 10, greater than motor normal frequency * 3
  DC bus Voltage Measurement Module : Subsystem  AncestorBlock=peripheral_utilities/Ideal Voltage Measurement with filter Module(ADC - Voltage)  mask{ADC_GAIN=DC_Voltage_Gain, ADC_BIT=ADC_Resolution, ADC_REFERENCE=DC_VOLTAGE_ADC_REFERENCE, ADC_BIAS=DC_VOLTAGE_ADC_BIAS, ADC_INIT=0, cut_frequency=DC_VOLTAGE_ADC_CUT_FREQ}
      mask DialogControl DescGroupVar Prompt: Voltage Sample ADC Model
      mask DialogControl DescTextVar Prompt: This is a ideal Voltage Measurement Module.
      mask DialogControl Control2 Prompt: ADC(p.u.) = (real_voltage * ADC_GAIN + ADC_BIAS)/ADC_REFERENCE
      mask DialogControl Control11 Prompt: GMP CTL Simulink Utilities: virtual peripherals
      mask DialogControl ParameterGroupVar Prompt: Parameters:
      mask DialogControl Control4 Prompt: ADC Voltage Gain (Scale Factor):
      mask DialogControl Control5 Prompt: ADC resolution:
      mask DialogControl Control6 Prompt: ADC reference Voltage(V)
      mask DialogControl Control8 Prompt: ADC Bias Voltage(V)
      mask DialogControl Control7 Prompt: ADC Initial Voltage Output (V):
      mask DialogControl Control9 Prompt: Voltage Filter cut frequency (Hz):
      mask DialogControl Control10 Prompt: Generally, this value less than switch frequency / 10, greater than motor normal frequency * 3
  DC/AC Half Bridge1 : gmp_peripheral_utilities/Single Phase Half Bridge (Duty Model)  fswitch=fswitch  CMP_MAX=CMP_MAX  Deadband_Upper=Deadband_Upper  Deadband_Lower=Deadband_Lower  Deadband_us=NaN  phase_shift=phase_shift  R_mosfet_on=R_mosfet_on  Lon=Lon  Rd=Rd  Vf=Vf  Rs=Rs  Cs=Cs
      settings: SourceProductName=Virtual Peripheral Utilities
  DC/AC Half Bridge2 : gmp_peripheral_utilities/Single Phase Half Bridge (Duty Model)  fswitch=fswitch  CMP_MAX=CMP_MAX  Deadband_Upper=Deadband_Upper  Deadband_Lower=Deadband_Lower  Deadband_us=NaN  phase_shift=phase_shift  R_mosfet_on=R_mosfet_on  Lon=Lon  Rd=Rd  Vf=Vf  Rs=Rs  Cs=Cs
      settings: SourceProductName=Virtual Peripheral Utilities
  Demux : Demux  Outputs=2
  Grid_Current_Sensor : spsSeriesRLCBranchLib/Series RLC Branch  LConnTagsString=__new0  RConnTagsString=__new0  BranchType=R  Resistance=GRID_CURRENT_SENSOR_R  Inductance=1e-3  SetiL0=off  InitialCurrent=0  Capacitance=1e-6  Setx0=off  InitialVoltage=0  Measurements=None
  Ideal Inductor Current Measurement Module（ADC - Current） : Subsystem  AncestorBlock=peripheral_utilities/Ideal Current Measurement Module（ADC - Current）  mask{ADC_GAIN=AC_Current_Gain, ADC_BIT=ADC_Resolution, ADC_REFERENCE=AC_CURRENT_ADC_REFERENCE, ADC_BIAS=AC_CURRENT_ADC_BIAS, ADC_INIT=AC_CURRENT_ADC_INIT}
      mask DialogControl DescGroupVar Prompt: Current Sample ADC Model 1
      mask DialogControl DescTextVar Prompt: This is a ideal Current Measurement Module. This module enable a bias and a gain, and finally output a ADC result.
      mask DialogControl Control8 Prompt: ADC(p.u.) = (real_current * ADC_GAIN + ADC_BIAS)/ADC_REFERENCE
      mask DialogControl Control9 Prompt: GMP CTL Simulink Utilities: virtual peripherals
      mask DialogControl ParameterGroupVar Prompt: 参数
      mask DialogControl Control7 Prompt: ADC Current Gain (Scale Factor):
      mask DialogControl Control2 Prompt: ADC resolution:
      mask DialogControl Control4 Prompt: ADC reference Current(A), ADC full scale current (when gain = 1)
      mask DialogControl Control5 Prompt: ADC Bias Current(A)
      mask DialogControl Control6 Prompt: ADC initial Current Output(A)
  Input_C : spsSeriesRLCBranchLib/Series RLC Branch  LConnTagsString=__new0  RConnTagsString=__new0  BranchType=RC  Resistance=DC_CAP_ESR  Inductance=1e-3  SetiL0=off  InitialCurrent=0  Capacitance=DC_CAP  Setx0=off  InitialVoltage=0  Measurements=None
  Input_C_EPR : spsSeriesRLCBranchLib/Series RLC Branch  LConnTagsString=__new0  RConnTagsString=__new0  BranchType=R  Resistance=DC_CAP_EPR  Inductance=1e-3  SetiL0=off  InitialCurrent=0  Capacitance=1e-6  Setx0=off  InitialVoltage=0  Measurements=None
  SINV_Current_Sensor : spsSeriesRLCBranchLib/Series RLC Branch  LConnTagsString=__new0  RConnTagsString=__new0  BranchType=R  Resistance=CAP_CURRENT_SENSOR_R  Inductance=1e-3  SetiL0=off  InitialCurrent=0  Capacitance=1e-6  Setx0=off  InitialVoltage=0  Measurements=None
  SINV_DC_BUS_Current_Sensor : spsSeriesRLCBranchLib/Series RLC Branch  LConnTagsString=__new0  RConnTagsString=__new0  BranchType=R  Resistance=DC_BUS_CURRENT_SENSOR_R  Inductance=1e-3  SetiL0=off  InitialCurrent=0  Capacitance=1e-6  Setx0=off  InitialVoltage=0  Measurements=None
  SINV_Filter_C : spsSeriesRLCBranchLib/Series RLC Branch  LConnTagsString=__new0  RConnTagsString=__new0  BranchType=RC  Resistance=ACF_C_ESR  Inductance=1e-3  SetiL0=off  InitialCurrent=0  Capacitance=ACF_C  Setx0=off  InitialVoltage=0  Measurements=None
  SINV_Filter_C_EPR : spsSeriesRLCBranchLib/Series RLC Branch  LConnTagsString=__new0  RConnTagsString=__new0  BranchType=R  Resistance=ACF_C_EPR  Inductance=1e-3  SetiL0=off  InitialCurrent=0  Capacitance=1e-6  Setx0=off  InitialVoltage=0  Measurements=None
  SINV_Filter_L : spsSeriesRLCBranchLib/Series RLC Branch  LConnTagsString=__new0  RConnTagsString=__new0  BranchType=RL  Resistance=ACF_L_ESR  Inductance=ACF_L  SetiL0=off  InitialCurrent=0  Capacitance=1e-6  Setx0=off  InitialVoltage=0  Measurements=None
  Scope{,1..2,8..17} (13 alike) : Scope
  Terminator3 : Terminator
  Voltage Measurement : spsVoltageMeasurementLib/Voltage Measurement  PhasorSimulation=off  OutputType=Complex  PSBequivalent=0
  DC_BUS+ : PMIOPort  Side=Left
  DC_BUS- : PMIOPort  Port=2  Side=Left
  AC_BUS_L : PMIOPort  Port=3  Side=Right
  AC_BUS_N : PMIOPort  Port=4  Side=Right
  ADC Port : Outport
  Trig : Outport  Port=2
  wires:
  Voltage Measurement/1 -> Scope/1
  [Sinv_IG] -> Bus Creator/6
  Capactor Current Measurement Module1/3(Sample & Hold View) -> Scope2/1
  Capactor Current Measurement Module1/2(Scope View (p.u.)) -> Scope1/1
  Capactor Current Measurement Module1/1(ADC OUT) -> [Sinv_IG]
  [SampleTrig] -> Capactor Current Measurement Module1/1(Sample Trigger)
  [SampleTrig] -> Trig/1
  Bus Creator/1 -> ADC Port/1
  [Sinv_VC] -> Bus Creator/5
  [Sinv_IC] -> Bus Creator/4
  [Sinv_IL] -> Bus Creator/1
  [Sinv_IDC] -> Bus Creator/2
  [Sinv_VDC] -> Bus Creator/3
  Demux/2 -> [BPWM2]
  Demux/1 -> [BPWM1]
  PWM CMP/1 -> Demux/1
  Enable/1 -> [EnableTag]
  DC Bus Current Measurement Module/1(ADC OUT) -> [Sinv_IDC]
  DC bus Voltage Measurement Module/1(ADC OUT) -> [Sinv_VDC]
  [SampleTrig] -> DC Bus Current Measurement Module/1(Sample Trigger)
  DC bus Voltage Measurement Module/3(Sample & Hold View) -> Scope15/1
  [BPWM1] -> DC/AC Half Bridge1/2
  DC Bus Current Measurement Module/3(Sample & Hold View) -> Scope17/1
  DC bus Voltage Measurement Module/2(Scope View (p.u.)) -> Scope14/1
  Ideal Inductor Current Measurement Module（ADC - Current）/2(Scope View (p.u.)) -> Scope12/1
  Ideal Inductor Current Measurement Module（ADC - Current）/1(ADC OUT) -> [Sinv_IL]
  DC Bus Current Measurement Module/2(Scope View (p.u.)) -> Scope16/1
  Ideal Inductor Current Measurement Module（ADC - Current）/3(Sample & Hold View) -> Scope13/1
  AC bus Voltage Measurement Module/1(ADC OUT) -> [Sinv_VC]
  Capactor Current Measurement Module/1(ADC OUT) -> [Sinv_IC]
  Capactor Current Measurement Module/2(Scope View (p.u.)) -> Scope10/1
  [SampleTrig] -> AC bus Voltage Measurement Module/1(Sample Trigger)
  [SampleTrig] -> Capactor Current Measurement Module/1(Sample Trigger)
  [EnableTag] -> DC/AC Half Bridge1/1
  Capactor Current Measurement Module/3(Sample & Hold View) -> Scope11/1
  [SampleTrig] -> DC bus Voltage Measurement Module/1(Sample Trigger)
  DC/AC Half Bridge1/1 -> Terminator3/1
  [EnableTag] -> DC/AC Half Bridge2/1
  AC bus Voltage Measurement Module/3(Sample & Hold View) -> Scope9/1
  AC bus Voltage Measurement Module/2(Scope View (p.u.)) -> Scope8/1
  [BPWM2] -> DC/AC Half Bridge2/2
  DC/AC Half Bridge2/1 -> [SampleTrig], Ideal Inductor Current Measurement Module（ADC - Current）/1(Sample Trigger)
  connections:
  DC/AC Half Bridge1/RConn1 -- SINV_Current_Sensor/RConn1 -- Grid_Current_Sensor/RConn1 -- Voltage Measurement/LConn2 -- AC bus Voltage Measurement Module/LConn2 -- Capactor Current Measurement Module1/LConn1 -- Capactor Current Measurement Module/LConn2
  DC/AC Half Bridge2/RConn1 -- Voltage Measurement/LConn1 -- Ideal Inductor Current Measurement Module（ADC - Current）/LConn1
  SINV_Filter_L/LConn1 -- Ideal Inductor Current Measurement Module（ADC - Current）/RConn1
  DC bus Voltage Measurement Module/LConn1 -- DC/AC Half Bridge2/LConn1 -- DC/AC Half Bridge1/LConn1 -- DC_BUS+/RConn1 -- Input_C/LConn1 -- Input_C_EPR/LConn1
  AC_BUS_N/RConn1 -- Capactor Current Measurement Module1/LConn2 -- Grid_Current_Sensor/LConn1
  Capactor Current Measurement Module/LConn1 -- SINV_Current_Sensor/LConn1 -- SINV_Filter_C_EPR/RConn1 -- SINV_Filter_C/RConn1
  DC bus Voltage Measurement Module/LConn2 -- DC/AC Half Bridge1/RConn2 -- SINV_DC_BUS_Current_Sensor/LConn1 -- DC/AC Half Bridge2/RConn2 -- DC Bus Current Measurement Module/LConn1
  DC Bus Current Measurement Module/LConn2 -- DC_BUS-/RConn1 -- Input_C/RConn1 -- Input_C_EPR/RConn1 -- SINV_DC_BUS_Current_Sensor/RConn1
  AC_BUS_L/RConn1 -- SINV_Filter_C_EPR/LConn1 -- SINV_Filter_L/RConn1 -- AC bus Voltage Measurement Module/LConn1 -- SINV_Filter_C/LConn1

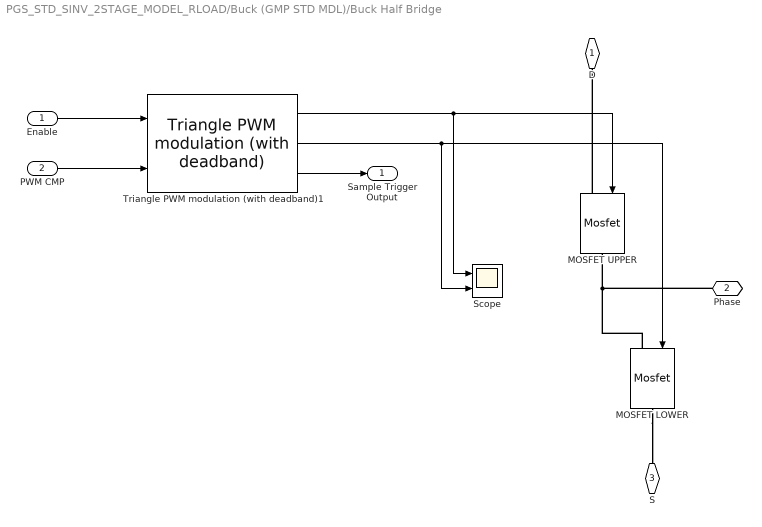
== system PGS_STD_SINV_2STAGE_MODEL_RLOAD/Buck (GMP STD MDL)/Buck Half Bridge ==
  Enable : Inport
  PWM CMP : Inport  Port=2
  MOSFET LOWER : spsMosfetLib/Mosfet  Ron=R_mosfet_on  Lon=Lon  Rd=Rd  Vfd=Vf  IC=0  Rs=Rs  Cs=Cs  Measurements=off
  MOSFET UPPER : spsMosfetLib/Mosfet  Ron=R_mosfet_on  Lon=Lon  Rd=Rd  Vfd=Vf  IC=0  Rs=Rs  Cs=Cs  Measurements=off
  Scope : Scope  NumInputPorts=2
  Triangle PWM modulation (with deadband)1 : gmp_fp_utilities/Triangle PWM modulation (with deadband)  fswitch=fswitch  CMP_MAX=CMP_MAX  Deadband_Upper=Deadband_Upper  Deadband_Lower=Deadband_Lower  phase_shift=phase_shift
      settings: SourceProductName=Fix-point Number Utilities
  D : PMIOPort  Side=Left
  Phase : PMIOPort  Port=2  Side=Right
  S : PMIOPort  Port=3  Side=Right
  Sample Trigger Output : Outport
  wires:
  Triangle PWM modulation (with deadband)1/1 -> MOSFET UPPER/1, Scope/1
  Enable/1 -> Triangle PWM modulation (with deadband)1/1
  Triangle PWM modulation (with deadband)1/3 -> Sample Trigger Output/1
  Triangle PWM modulation (with deadband)1/2 -> MOSFET LOWER/1, Scope/2
  PWM CMP/1 -> Triangle PWM modulation (with deadband)1/2
  connections:
  MOSFET UPPER/LConn1 -- D/RConn1
  MOSFET LOWER/LConn1 -- Phase/RConn1 -- MOSFET UPPER/RConn1
  MOSFET LOWER/RConn1 -- S/RConn1
